simulink model "Model_1_0_simple"  (R2019b)
settings: Solver=VariableStepAuto  StartTime=0.0  StopTime=100.0  RelTol=1e-3
undefined symbols (not defined in the file or in its folder): alpha_E, alpha_I, beta_C, beta_E, beta_H, beta_I, delta_E, delta_I, delta_S, eta, gamma_C, gamma_E, gamma_I, gamma_R, gamma_S, mu, rho, xi
settings Model: Creator=Pål  LastModifiedBy=Pål

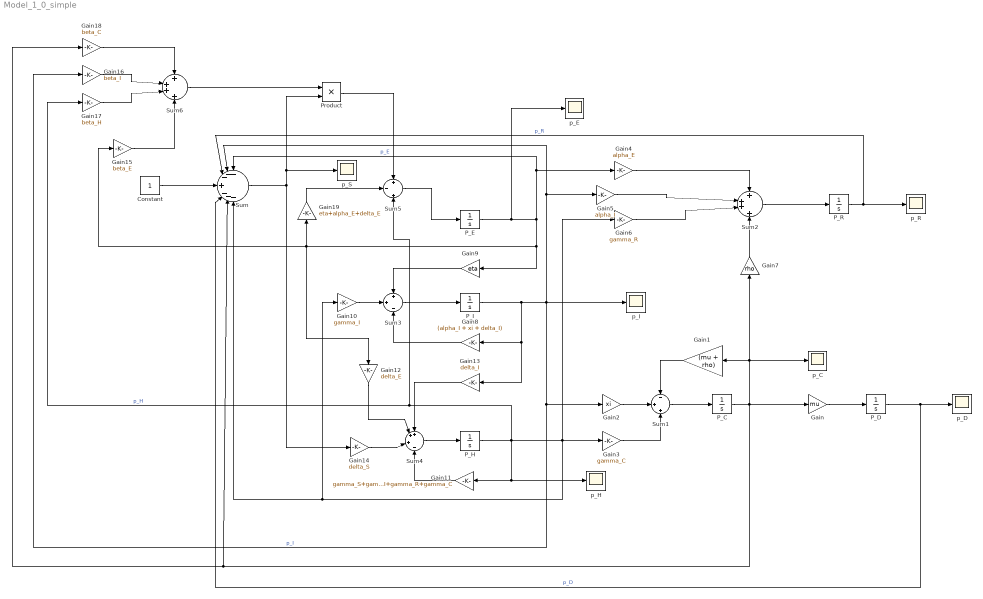
== system Model_1_0_simple ==
  Constant : Constant
  Gain : Gain  Gain=mu
  Gain1 : Gain  Gain=(mu + rho)
  Gain10 : Gain  Gain=gamma_I
  Gain11 : Gain  Gain=gamma_S+gamma_E+gamma_I+gamma_R+gamma_C
  Gain12 : Gain  Gain=delta_E
  Gain13 : Gain  Gain=delta_I
  Gain14 : Gain  Gain=delta_S
  Gain15 : Gain  Gain=beta_E
  Gain16 : Gain  Gain=beta_I
  Gain17 : Gain  Gain=beta_H
  Gain18 : Gain  Gain=beta_C
  Gain19 : Gain  Gain=eta+alpha_E+delta_E
  Gain2 : Gain  Gain=xi
  Gain3 : Gain  Gain=gamma_C
  Gain4 : Gain  Gain=alpha_E
  Gain5 : Gain  Gain=alpha_I
  Gain6 : Gain  Gain=gamma_R
  Gain7 : Gain  Gain=rho
  Gain8 : Gain  Gain=(alpha_I + xi + delta_I)
  Gain9 : Gain  Gain=eta
  P_C : Integrator  InitialCondition=[0]
  P_D : Integrator  InitialCondition=[0]
  P_E : Integrator  InitialCondition=[0.000025]
  P_H : Integrator  InitialCondition=[0]
  P_I : Integrator  InitialCondition=[0]
  P_R : Integrator  InitialCondition=[0]
  Product : Product
  Sum : Sum  Inputs=---|+|---
  Sum1 : Sum  Inputs=-|+|+
  Sum2 : Sum  Inputs=+|++|+
  Sum3 : Sum  Inputs=+|+|-
  Sum4 : Sum  Inputs=++|+|-
  Sum5 : Sum  Inputs=+|-|+
  Sum6 : Sum  Inputs=+|++|+
  p_C : Scope
  "p_D " : Scope
  p_E : Scope
  p_H : Scope
  p_I : Scope
  p_R : Scope
  "p_S " : Scope
  wires:
  P_C/1 -> p_C/1, Gain7/1, Gain1/1, Sum/6, Gain18/1, Gain/1
  Gain/1 -> P_D/1
  Sum1/1 -> P_C/1
  Gain1/1 -> Sum1/1
  P_H/1 -> Gain11/1, p_H/1, Gain17/1, Sum5/3, Gain6/1, Sum/7, Gain10/1, Gain3/1  "p_H"
  Gain3/1 -> Sum1/3
  Gain2/1 -> Sum1/2
  P_I/1 -> p_I/1, Gain16/1, Gain2/1, Gain5/1, Sum/2, Gain13/1, Gain8/1  "p_I"
  Sum2/1 -> P_R/1
  P_E/1 -> p_E/1, Sum/1, Gain4/1, Gain12/1, Gain19/1, Gain15/1, Gain9/1  "p_E"
  Gain4/1 -> Sum2/1
  Gain5/1 -> Sum2/2
  Gain6/1 -> Sum2/3
  Gain7/1 -> Sum2/4
  Sum3/1 -> P_I/1
  Gain8/1 -> Sum3/3
  Gain9/1 -> Sum3/1
  Gain10/1 -> Sum3/2
  Sum4/1 -> P_H/1
  Gain11/1 -> Sum4/4
  Gain12/1 -> Sum4/2
  Gain13/1 -> Sum4/1
  Sum/1 -> "p_S "/1, Product/2, Gain14/1
  Gain14/1 -> Sum4/3
  Sum5/1 -> P_E/1
  Sum6/1 -> Product/1
  Product/1 -> Sum5/1
  Gain18/1 -> Sum6/1
  Gain16/1 -> Sum6/2
  Gain17/1 -> Sum6/3
  Gain15/1 -> Sum6/4
  Gain19/1 -> Sum5/2
  P_R/1 -> p_R/1, Sum/3  "p_R"
  Constant/1 -> Sum/4
  P_D/1 -> "p_D "/1, Sum/5  "p_D"
